simulink model "lab_10_4_2018"  (R2018a)
settings: Solver=VariableStepAuto  StartTime=0.0  StopTime=10.0  RelTol=1e-3
undefined symbols (not defined in the file): A, B, C, Continuous, D, K, Time
libraries: ctrlSharedLib x1
settings Model: Creator=osini  LastModifiedBy=osini
settings DataIOCC: ReturnWorkspaceOutputs=on
settings DebuggingCC: UnconnectedInputMsg=none  UnconnectedOutputMsg=none  UnconnectedLineMsg=none  SFMachineParentedDataDiag=error
settings ModelReferenceCC: EnableRefExpFcnMdlSchedulingChecks=off
settings SFSimCC: SimUseLocalCustomCode=on
settings RTWCC: Description=Generic Real-Time Target  RTWUseLocalCustomCode=on

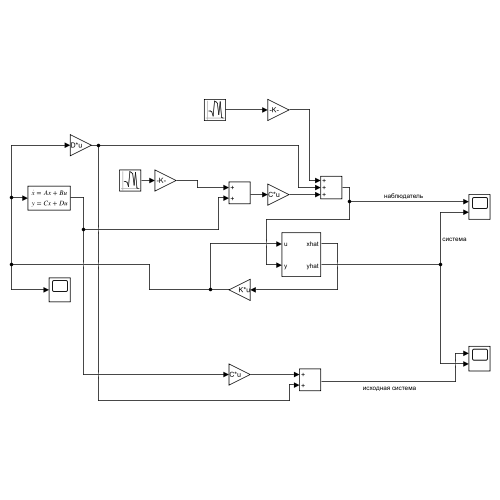
[thumbnail: Simulink's stored preview of the top-level diagram]
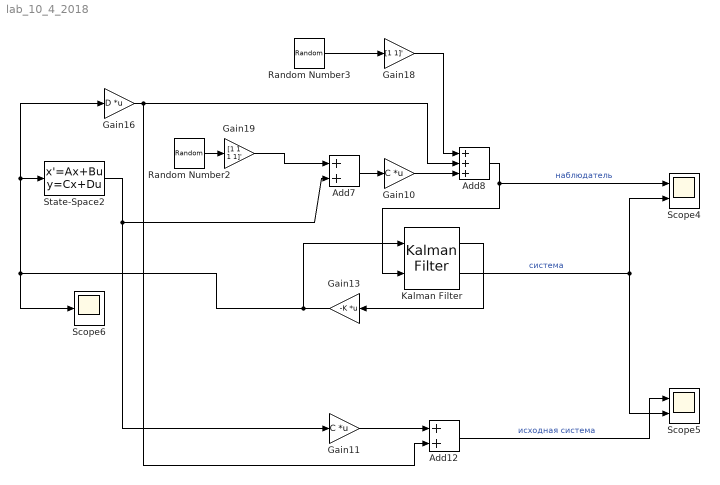
== system lab_10_4_2018 ==
  Add12 : Sum
  Add7 : Sum
  Add8 : Sum  Inputs=+++
  Gain10 : Gain  Gain=C  Multiplication=Matrix(K*u)
  Gain11 : Gain  Gain=C  Multiplication=Matrix(K*u)
  Gain13 : Gain  Gain=-K  Multiplication=Matrix(K*u)
  Gain16 : Gain  Gain=D  Multiplication=Matrix(K*u)
  Gain18 : Gain  Gain=[1 1]'
  Gain19 : Gain  Gain=[1 1 1 1]'
  Kalman Filter : ctrlSharedLib/Kalman Filter  TimeDomain=Continuous-Time  UseCurrentEstimator=on  ModelSource=Individual A, B, C, D matrices  ModelSourceVariable=ss(0.95,1,1,0,1)  A=A  B=B  C=C  D=D  NumberOfStates=1  NumberOfInputs=1  NumberOfOutputs=1  InitialEstimateSource=Dialog  X0=[4 3 2 1]  P0=10  UseK=off  UseGH=off  NumberOfProcessNoiseInputs=1  G=zeros(4,4)  TimeInvariantG=on  H=0  TimeInvariantH=on  Q=250  TimeInvariantQ=on  R=5  TimeInvariantR=on  N=0  TimeInvariantN=on  AddInputPort=on  AddEnablePort=off  OutputEstimatedY=on  OutputP=off  Ts=-1
  Random Number2 : RandomNumber  Variance=250  SampleTime=0.1
  Random Number3 : RandomNumber  Variance=5  SampleTime=0.1
  Scope4 : Scope  NumInputPorts=2
  Scope5 : Scope  NumInputPorts=2
  Scope6 : Scope
  State-Space2 : StateSpace  A=A  B=B  C=eye(4,4)  D=zeros(4, 2)  InitialCondition=[1]
  wires:
  Add12/1 -> Scope5/1  "исходная система"
  Kalman Filter/1 -> Gain13/1
  Gain16/1 -> Add8/2, Add12/2
  Gain10/1 -> Add8/3
  Add7/1 -> Gain10/1
  Gain13/1 -> Kalman Filter/1, Scope6/1, Gain16/1, State-Space2/1
  Gain11/1 -> Add12/1
  State-Space2/1 -> Add7/2, Gain11/1
  Add8/1 -> Scope4/1, Kalman Filter/2  "наблюдатель"
  Kalman Filter/2 -> Scope4/2, Scope5/2  "система"
  Random Number3/1 -> Gain18/1
  Gain18/1 -> Add8/1
  Gain19/1 -> Add7/1
  Random Number2/1 -> Gain19/1
